simulink model "PACING_CIRCUIT_TEST"  (R2020b)
settings: Solver=FixedStepAuto  StartTime=0.0  StopTime=5.0  FixedStep=1e-3  RelTol=1e-3  EnableMultiTasking=on
undefined symbols (not defined in the file): D10, D11, D12, D2, D4, D5, D7, D8, D9, PTA0, PTA2, PTB23, PTB9, PTC3, PTC4, PTD0, PTD2, PTD3
libraries: frdmk64flib x12
settings Model: ExtModeTrigDuration=5  Creator=Daniyal  LastModifiedBy=Nour
settings OptimizationCC: EnhancedBackFolding=on  PassReuseOutputArgsAs=Individual arguments  ZeroExternalMemoryAtStartup=off  ZeroInternalMemoryAtStartup=off  MaxStackSize=64  OptimizeBlockOrder=speed  DifferentSizesBufferReuse=on  OptimizationCustomize=off  EfficientTunableParamExpr=on
settings DebuggingCC: ParameterTunabilityLossMsg=error
settings HardwareCC: ProdBitPerPointer=32  ProdBitPerSizeT=32  ProdBitPerPtrDiffT=32  ProdLargestAtomicInteger=Long  ProdLargestAtomicFloat=Double  ProdWordSize=32  ProdHWDeviceType=ARM Compatible->ARM Cortex
settings SFSimCC: MATLABDynamicMemAlloc=off
settings RTWCC: Description=Embedded Coder  SystemTargetFile=ert.tlc  HardwareBoard=NXP FRDM-K64F  TLCOptions="-aInlineSetEventsForThisBaseRateFcn=TLC_FALSE -aSuppressMultiTaskScheduler=TLC_FALSE  -aRateBasedStepFcn=0"  TemplateMakefile=ert_default_tmf  Toolchain=GNU Tools for ARM Embedded Processors
settings CodeAppCC: ForceParamTrailComments=on  IgnoreCustomStorageClasses=off  OperatorAnnotations=on  SimulinkDataObjDesc=on  SFDataObjDesc=on  InsertBlockDesc=on

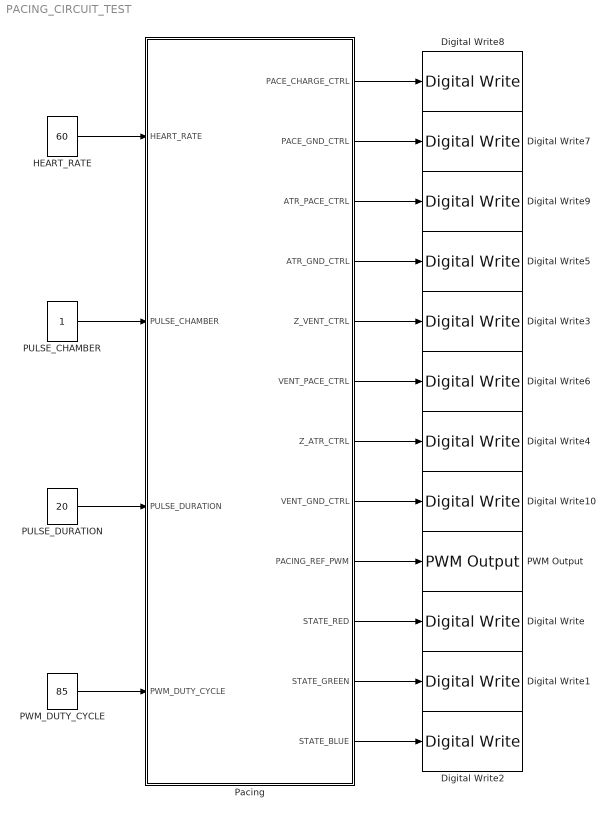
== system PACING_CIRCUIT_TEST ==
  Digital Write : frdmk64flib/Digital Write  Whichpin=RED_LED
  Digital Write1 : frdmk64flib/Digital Write  Whichpin=GREEN_LED
  Digital Write10 : frdmk64flib/Digital Write  Whichpin=PTD3 (D12)
  Digital Write2 : frdmk64flib/Digital Write  Whichpin=BLUE_LED
  Digital Write3 : frdmk64flib/Digital Write  Whichpin=PTC3 (D7)
  Digital Write4 : frdmk64flib/Digital Write  Whichpin=PTB23 (D4)
  Digital Write5 : frdmk64flib/Digital Write  Whichpin=PTD2 (D11)
  Digital Write6 : frdmk64flib/Digital Write  Whichpin=PTC4 (D9)
  Digital Write7 : frdmk64flib/Digital Write  Whichpin=PTD0 (D10)
  Digital Write8 : frdmk64flib/Digital Write  Whichpin=PTB9 (D2)
  Digital Write9 : frdmk64flib/Digital Write  Whichpin=PTA0 (D8)
  HEART_RATE : Constant  Value=60
  PULSE_CHAMBER : Constant
  PULSE_DURATION : Constant  Value=20
  PWM Output : frdmk64flib/PWM Output  Whichpin=PTA2 (D5)  InitialFrequency=2000  InitialDutyCycle=85
  PWM_DUTY_CYCLE : Constant  Value=85
  Pacing : Stateflow chart  TreatAsAtomicUnit=on
  wires:
  HEART_RATE/1 -> Pacing/1(HEART_RATE)
  PWM_DUTY_CYCLE/1 -> Pacing/4(PWM_DUTY_CYCLE)
  PULSE_CHAMBER/1 -> Pacing/2(PULSE_CHAMBER)
  PULSE_DURATION/1 -> Pacing/3(PULSE_DURATION)
  Pacing/12(STATE_BLUE) -> Digital Write2/1
  Pacing/11(STATE_GREEN) -> Digital Write1/1
  Pacing/10(STATE_RED) -> Digital Write/1
  Pacing/9(PACING_REF_PWM) -> PWM Output/1
  Pacing/8(VENT_GND_CTRL) -> Digital Write10/1
  Pacing/7(Z_ATR_CTRL) -> Digital Write4/1
  Pacing/6(VENT_PACE_CTRL) -> Digital Write6/1
  Pacing/5(Z_VENT_CTRL) -> Digital Write3/1
  Pacing/4(ATR_GND_CTRL) -> Digital Write5/1
  Pacing/3(ATR_PACE_CTRL) -> Digital Write9/1
  Pacing/2(PACE_GND_CTRL) -> Digital Write7/1
  Pacing/1(PACE_CHARGE_CTRL) -> Digital Write8/1

== stateflow chart PACING_CIRCUIT_TEST/Pacing ==
  state PULSE_ATRIUM
    %% PULSE_CHAMBER == 1 is for Atr
    entry:
    during:
    STATE_RED = 0;
    STATE_GREEN = 0;
    STATE_BLUE = 1;
    PACE_CHARGE_CTRL =  false;
    PACE_GND_CTRL = true;
    ATR_PACE_CTRL = true;
    ATR_GND_CTRL =  false;
    Z_ATR_CTRL = false;
    Z_VENT_CTRL =  false;
    VENT_GND_CTRL =false;
    VENT_PACE_CTRL =  false;
    exit:
  state CHARGE
    entry:
    during:
    STATE_RED = 1;
    STATE_GREEN = 0;
    STATE_BLUE = 0;
    ATR_PACE_CTRL = false;
    VENT_PACE_CTRL  = false;
    PACING_REF_PWM = PWM_DUTY_CYCLE;
    PACE_CHARGE_CTRL = true;
    PACE_GND_CTRL = true;
    VENT_PACE_CTRL = false;
    Z_ATR_CTRL =  false;
    Z_VENT_CTRL =  false;
    ATR_PACE_CTRL =  false;
    if (PULSE_CHAMBER==1)
    ATR_GND_CTRL = true;
    VENT_GND_CTRL =  false;
    else
    ATR_GND_CTRL = false;
    VENT_GND_CTRL = true;
    end
    exit:
  state PULSE_VENTRICLE
    %% PULSE_CHAMBER == 2 is for VENT
    entry:
    during:
    STATE_RED = 0;
    STATE_GREEN = 1;
    STATE_BLUE = 0;
    PACE_CHARGE_CTRL =  false;
    PACE_GND_CTRL = true;
    ATR_PACE_CTRL = false;
    ATR_GND_CTRL =  false;
    Z_ATR_CTRL = false;
    Z_VENT_CTRL =  false;
    VENT_GND_CTRL =false;
    VENT_PACE_CTRL =  true;
    exit:
  CHARGE -> PULSE_ATRIUM [order 1] : [[after((60000/HEART_RATE)-PULSE_DURATION,msec) & (PULSE_CHAMBER==1) ]]
  (default) -> CHARGE
  PULSE_ATRIUM -> CHARGE : [after(PULSE_DURATION,msec)]
  PULSE_VENTRICLE -> CHARGE : [after(PULSE_DURATION,msec)]
  CHARGE -> PULSE_VENTRICLE [order 2] : [[after((60000/HEART_RATE)-PULSE_DURATION, msec) & (PULSE_CHAMBER==2) ]]
  data: HEART_RATE input double; PULSE_CHAMBER input double; PULSE_DURATION input double; PWM_DUTY_CYCLE input double; PACE_CHARGE_CTRL output boolean =false; PACE_GND_CTRL output boolean =false; ATR_PACE_CTRL output boolean =false; ATR_GND_CTRL output boolean =false; Z_VENT_CTRL output boolean =false; VENT_PACE_CTRL output boolean =false; Z_ATR_CTRL output boolean =false; VENT_GND_CTRL output boolean =false; PACING_REF_PWM output double; STATE_RED output int16; STATE_GREEN output int16; STATE_BLUE output int16
